simulink model "UberSpurs"  (R2015b)
settings: Solver=VariableStepAuto  StartTime=0.0  StopTime=5000  RelTol=1e-3
libraries: simulink x54
(part 5 of 6)

== system UberSpurs/spur3WorkCell/route2Channel16 ==
  serverAvailable : Inport
  Constant : Constant  Value=16
  Get Attribute : GetAttribute  AttributeName=Channel|FillTime  AttributeMissing=Error|Error  AttributeDefaultValue=1|1  AttributeTreatAsVector=1|1  AttributeSendTiming=After entity departure|After entity departure  EvaluatedDefaultAttributeValue={ [];[]}
      settings: OutputPortMap=o1,o2
  RoutingControlActuator : OutputSwitch  NumberOutputPorts=2  SwitchingCriterion=From signal port p  InitialConditionsOpt=on
  RoutingControlBehavior : Stateflow chart  TreatAsAtomicUnit=on
  Single Server1 : SingleServer  ServiceTime=0
  toChannel : PMIOPort  Port=1  Side=Right
  fromMHS : PMIOPort  Port=2  Side=Left
  toMHS : PMIOPort  Port=3  Side=Right
  wires:
  RoutingControlBehavior/1(route) -> RoutingControlActuator/1
  Constant/1 -> RoutingControlBehavior/2(channel)
  Get Attribute/1 -> RoutingControlBehavior/1(entityChannel)
  serverAvailable/1 -> RoutingControlBehavior/3(serverAvailable)
  Get Attribute/2 -> RoutingControlBehavior/4(FillTime)
  connections:
  RoutingControlActuator/RConn2 -- toMHS/RConn1
  Get Attribute/RConn1 -- Single Server1/LConn1
  fromMHS/RConn1 -- Get Attribute/LConn1
  toChannel/RConn1 -- RoutingControlActuator/RConn1
  Single Server1/RConn1 -- RoutingControlActuator/LConn1

== system UberSpurs/spur3WorkCell/route2Channel17 ==
  serverAvailable : Inport
  Constant : Constant  Value=17
  Get Attribute : GetAttribute  AttributeName=Channel|FillTime  AttributeMissing=Error|Error  AttributeDefaultValue=1|1  AttributeTreatAsVector=1|1  AttributeSendTiming=After entity departure|After entity departure  EvaluatedDefaultAttributeValue={ [];[]}
      settings: OutputPortMap=o1,o2
  RoutingControlActuator : OutputSwitch  NumberOutputPorts=2  SwitchingCriterion=From signal port p  InitialConditionsOpt=on
  RoutingControlBehavior : Stateflow chart  TreatAsAtomicUnit=on
  Single Server1 : SingleServer  ServiceTime=0
  toChannel : PMIOPort  Port=1  Side=Right
  fromMHS : PMIOPort  Port=2  Side=Left
  toMHS : PMIOPort  Port=3  Side=Right
  wires:
  RoutingControlBehavior/1(route) -> RoutingControlActuator/1
  Constant/1 -> RoutingControlBehavior/2(channel)
  Get Attribute/1 -> RoutingControlBehavior/1(entityChannel)
  serverAvailable/1 -> RoutingControlBehavior/3(serverAvailable)
  Get Attribute/2 -> RoutingControlBehavior/4(FillTime)
  connections:
  RoutingControlActuator/RConn2 -- toMHS/RConn1
  Get Attribute/RConn1 -- Single Server1/LConn1
  fromMHS/RConn1 -- Get Attribute/LConn1
  toChannel/RConn1 -- RoutingControlActuator/RConn1
  Single Server1/RConn1 -- RoutingControlActuator/LConn1

== system UberSpurs/spur3WorkCell/route2Channel18 ==
  serverAvailable : Inport
  Constant : Constant  Value=18
  Get Attribute : GetAttribute  AttributeName=Channel|FillTime  AttributeMissing=Error|Error  AttributeDefaultValue=1|1  AttributeTreatAsVector=1|1  AttributeSendTiming=After entity departure|After entity departure  EvaluatedDefaultAttributeValue={ [];[]}
      settings: OutputPortMap=o1,o2
  RoutingControlActuator : OutputSwitch  NumberOutputPorts=2  SwitchingCriterion=From signal port p  InitialConditionsOpt=on
  RoutingControlBehavior : Stateflow chart  TreatAsAtomicUnit=on
  Single Server1 : SingleServer  ServiceTime=0
  toChannel : PMIOPort  Port=1  Side=Right
  fromMHS : PMIOPort  Port=2  Side=Left
  toMHS : PMIOPort  Port=3  Side=Right
  wires:
  RoutingControlBehavior/1(route) -> RoutingControlActuator/1
  Constant/1 -> RoutingControlBehavior/2(channel)
  Get Attribute/1 -> RoutingControlBehavior/1(entityChannel)
  serverAvailable/1 -> RoutingControlBehavior/3(serverAvailable)
  Get Attribute/2 -> RoutingControlBehavior/4(FillTime)
  connections:
  RoutingControlActuator/RConn2 -- toMHS/RConn1
  Get Attribute/RConn1 -- Single Server1/LConn1
  fromMHS/RConn1 -- Get Attribute/LConn1
  toChannel/RConn1 -- RoutingControlActuator/RConn1
  Single Server1/RConn1 -- RoutingControlActuator/LConn1

== system UberSpurs/spur3WorkCell/route2Channel2 ==
  serverAvailable : Inport
  Constant : Constant  Value=2
  Get Attribute : GetAttribute  AttributeName=Channel|FillTime  AttributeMissing=Error|Error  AttributeDefaultValue=1|1  AttributeTreatAsVector=1|1  AttributeSendTiming=After entity departure|After entity departure  EvaluatedDefaultAttributeValue={ [];[]}
      settings: OutputPortMap=o1,o2
  RoutingControlActuator : OutputSwitch  NumberOutputPorts=2  SwitchingCriterion=From signal port p  InitialConditionsOpt=on
  RoutingControlBehavior : Stateflow chart  TreatAsAtomicUnit=on
  Single Server1 : SingleServer  ServiceTime=0
  toChannel : PMIOPort  Port=1  Side=Right
  fromMHS : PMIOPort  Port=2  Side=Left
  toMHS : PMIOPort  Port=3  Side=Right
  wires:
  RoutingControlBehavior/1(route) -> RoutingControlActuator/1
  Constant/1 -> RoutingControlBehavior/2(channel)
  Get Attribute/1 -> RoutingControlBehavior/1(entityChannel)
  serverAvailable/1 -> RoutingControlBehavior/3(serverAvailable)
  Get Attribute/2 -> RoutingControlBehavior/4(FillTime)
  connections:
  RoutingControlActuator/RConn2 -- toMHS/RConn1
  Get Attribute/RConn1 -- Single Server1/LConn1
  fromMHS/RConn1 -- Get Attribute/LConn1
  toChannel/RConn1 -- RoutingControlActuator/RConn1
  Single Server1/RConn1 -- RoutingControlActuator/LConn1

== system UberSpurs/spur3WorkCell/route2Channel3 ==
  serverAvailable : Inport
  Constant : Constant  Value=3
  Get Attribute : GetAttribute  AttributeName=Channel|FillTime  AttributeMissing=Error|Error  AttributeDefaultValue=1|1  AttributeTreatAsVector=1|1  AttributeSendTiming=After entity departure|After entity departure  EvaluatedDefaultAttributeValue={ [];[]}
      settings: OutputPortMap=o1,o2
  RoutingControlActuator : OutputSwitch  NumberOutputPorts=2  SwitchingCriterion=From signal port p  InitialConditionsOpt=on
  RoutingControlBehavior : Stateflow chart  TreatAsAtomicUnit=on
  Single Server1 : SingleServer  ServiceTime=0
  toChannel : PMIOPort  Port=1  Side=Right
  fromMHS : PMIOPort  Port=2  Side=Left
  toMHS : PMIOPort  Port=3  Side=Right
  wires:
  RoutingControlBehavior/1(route) -> RoutingControlActuator/1
  Constant/1 -> RoutingControlBehavior/2(channel)
  Get Attribute/1 -> RoutingControlBehavior/1(entityChannel)
  serverAvailable/1 -> RoutingControlBehavior/3(serverAvailable)
  Get Attribute/2 -> RoutingControlBehavior/4(FillTime)
  connections:
  RoutingControlActuator/RConn2 -- toMHS/RConn1
  Get Attribute/RConn1 -- Single Server1/LConn1
  fromMHS/RConn1 -- Get Attribute/LConn1
  toChannel/RConn1 -- RoutingControlActuator/RConn1
  Single Server1/RConn1 -- RoutingControlActuator/LConn1

== system UberSpurs/spur3WorkCell/route2Channel4 ==
  serverAvailable : Inport
  Constant : Constant  Value=4
  Get Attribute : GetAttribute  AttributeName=Channel|FillTime  AttributeMissing=Error|Error  AttributeDefaultValue=1|1  AttributeTreatAsVector=1|1  AttributeSendTiming=After entity departure|After entity departure  EvaluatedDefaultAttributeValue={ [];[]}
      settings: OutputPortMap=o1,o2
  RoutingControlActuator : OutputSwitch  NumberOutputPorts=2  SwitchingCriterion=From signal port p  InitialConditionsOpt=on
  RoutingControlBehavior : Stateflow chart  TreatAsAtomicUnit=on
  Single Server1 : SingleServer  ServiceTime=0
  toChannel : PMIOPort  Port=1  Side=Right
  fromMHS : PMIOPort  Port=2  Side=Left
  toMHS : PMIOPort  Port=3  Side=Right
  wires:
  RoutingControlBehavior/1(route) -> RoutingControlActuator/1
  Constant/1 -> RoutingControlBehavior/2(channel)
  Get Attribute/1 -> RoutingControlBehavior/1(entityChannel)
  serverAvailable/1 -> RoutingControlBehavior/3(serverAvailable)
  Get Attribute/2 -> RoutingControlBehavior/4(FillTime)
  connections:
  RoutingControlActuator/RConn2 -- toMHS/RConn1
  Get Attribute/RConn1 -- Single Server1/LConn1
  fromMHS/RConn1 -- Get Attribute/LConn1
  toChannel/RConn1 -- RoutingControlActuator/RConn1
  Single Server1/RConn1 -- RoutingControlActuator/LConn1

== system UberSpurs/spur3WorkCell/route2Channel5 ==
  serverAvailable : Inport
  Constant : Constant  Value=5
  Get Attribute : GetAttribute  AttributeName=Channel|FillTime  AttributeMissing=Error|Error  AttributeDefaultValue=1|1  AttributeTreatAsVector=1|1  AttributeSendTiming=After entity departure|After entity departure  EvaluatedDefaultAttributeValue={ [];[]}
      settings: OutputPortMap=o1,o2
  RoutingControlActuator : OutputSwitch  NumberOutputPorts=2  SwitchingCriterion=From signal port p  InitialConditionsOpt=on
  RoutingControlBehavior : Stateflow chart  TreatAsAtomicUnit=on
  Single Server1 : SingleServer  ServiceTime=0
  toChannel : PMIOPort  Port=1  Side=Right
  fromMHS : PMIOPort  Port=2  Side=Left
  toMHS : PMIOPort  Port=3  Side=Right
  wires:
  RoutingControlBehavior/1(route) -> RoutingControlActuator/1
  Constant/1 -> RoutingControlBehavior/2(channel)
  Get Attribute/1 -> RoutingControlBehavior/1(entityChannel)
  serverAvailable/1 -> RoutingControlBehavior/3(serverAvailable)
  Get Attribute/2 -> RoutingControlBehavior/4(FillTime)
  connections:
  RoutingControlActuator/RConn2 -- toMHS/RConn1
  Get Attribute/RConn1 -- Single Server1/LConn1
  fromMHS/RConn1 -- Get Attribute/LConn1
  toChannel/RConn1 -- RoutingControlActuator/RConn1
  Single Server1/RConn1 -- RoutingControlActuator/LConn1

== system UberSpurs/spur3WorkCell/route2Channel6 ==
  serverAvailable : Inport
  Constant : Constant  Value=6
  Get Attribute : GetAttribute  AttributeName=Channel|FillTime  AttributeMissing=Error|Error  AttributeDefaultValue=1|1  AttributeTreatAsVector=1|1  AttributeSendTiming=After entity departure|After entity departure  EvaluatedDefaultAttributeValue={ [];[]}
      settings: OutputPortMap=o1,o2
  RoutingControlActuator : OutputSwitch  NumberOutputPorts=2  SwitchingCriterion=From signal port p  InitialConditionsOpt=on
  RoutingControlBehavior : Stateflow chart  TreatAsAtomicUnit=on
  Single Server1 : SingleServer  ServiceTime=0
  toChannel : PMIOPort  Port=1  Side=Right
  fromMHS : PMIOPort  Port=2  Side=Left
  toMHS : PMIOPort  Port=3  Side=Right
  wires:
  RoutingControlBehavior/1(route) -> RoutingControlActuator/1
  Constant/1 -> RoutingControlBehavior/2(channel)
  Get Attribute/1 -> RoutingControlBehavior/1(entityChannel)
  serverAvailable/1 -> RoutingControlBehavior/3(serverAvailable)
  Get Attribute/2 -> RoutingControlBehavior/4(FillTime)
  connections:
  RoutingControlActuator/RConn2 -- toMHS/RConn1
  Get Attribute/RConn1 -- Single Server1/LConn1
  fromMHS/RConn1 -- Get Attribute/LConn1
  toChannel/RConn1 -- RoutingControlActuator/RConn1
  Single Server1/RConn1 -- RoutingControlActuator/LConn1

== system UberSpurs/spur3WorkCell/route2Channel7 ==
  serverAvailable : Inport
  Constant : Constant  Value=7
  Get Attribute : GetAttribute  AttributeName=Channel|FillTime  AttributeMissing=Error|Error  AttributeDefaultValue=1|1  AttributeTreatAsVector=1|1  AttributeSendTiming=After entity departure|After entity departure  EvaluatedDefaultAttributeValue={ [];[]}
      settings: OutputPortMap=o1,o2
  RoutingControlActuator : OutputSwitch  NumberOutputPorts=2  SwitchingCriterion=From signal port p  InitialConditionsOpt=on
  RoutingControlBehavior : Stateflow chart  TreatAsAtomicUnit=on
  Single Server1 : SingleServer  ServiceTime=0
  toChannel : PMIOPort  Port=1  Side=Right
  fromMHS : PMIOPort  Port=2  Side=Left
  toMHS : PMIOPort  Port=3  Side=Right
  wires:
  RoutingControlBehavior/1(route) -> RoutingControlActuator/1
  Constant/1 -> RoutingControlBehavior/2(channel)
  Get Attribute/1 -> RoutingControlBehavior/1(entityChannel)
  serverAvailable/1 -> RoutingControlBehavior/3(serverAvailable)
  Get Attribute/2 -> RoutingControlBehavior/4(FillTime)
  connections:
  RoutingControlActuator/RConn2 -- toMHS/RConn1
  Get Attribute/RConn1 -- Single Server1/LConn1
  fromMHS/RConn1 -- Get Attribute/LConn1
  toChannel/RConn1 -- RoutingControlActuator/RConn1
  Single Server1/RConn1 -- RoutingControlActuator/LConn1

== system UberSpurs/spur3WorkCell/route2Channel8 ==
  serverAvailable : Inport
  Constant : Constant  Value=8
  Get Attribute : GetAttribute  AttributeName=Channel|FillTime  AttributeMissing=Error|Error  AttributeDefaultValue=1|1  AttributeTreatAsVector=1|1  AttributeSendTiming=After entity departure|After entity departure  EvaluatedDefaultAttributeValue={ [];[]}
      settings: OutputPortMap=o1,o2
  RoutingControlActuator : OutputSwitch  NumberOutputPorts=2  SwitchingCriterion=From signal port p  InitialConditionsOpt=on
  RoutingControlBehavior : Stateflow chart  TreatAsAtomicUnit=on
  Single Server1 : SingleServer  ServiceTime=0
  toChannel : PMIOPort  Port=1  Side=Right
  fromMHS : PMIOPort  Port=2  Side=Left
  toMHS : PMIOPort  Port=3  Side=Right
  wires:
  RoutingControlBehavior/1(route) -> RoutingControlActuator/1
  Constant/1 -> RoutingControlBehavior/2(channel)
  Get Attribute/1 -> RoutingControlBehavior/1(entityChannel)
  serverAvailable/1 -> RoutingControlBehavior/3(serverAvailable)
  Get Attribute/2 -> RoutingControlBehavior/4(FillTime)
  connections:
  RoutingControlActuator/RConn2 -- toMHS/RConn1
  Get Attribute/RConn1 -- Single Server1/LConn1
  fromMHS/RConn1 -- Get Attribute/LConn1
  toChannel/RConn1 -- RoutingControlActuator/RConn1
  Single Server1/RConn1 -- RoutingControlActuator/LConn1

== system UberSpurs/spur3WorkCell/route2Channel9 ==
  serverAvailable : Inport
  Constant : Constant  Value=9
  Get Attribute : GetAttribute  AttributeName=Channel|FillTime  AttributeMissing=Error|Error  AttributeDefaultValue=1|1  AttributeTreatAsVector=1|1  AttributeSendTiming=After entity departure|After entity departure  EvaluatedDefaultAttributeValue={ [];[]}
      settings: OutputPortMap=o1,o2
  RoutingControlActuator : OutputSwitch  NumberOutputPorts=2  SwitchingCriterion=From signal port p  InitialConditionsOpt=on
  RoutingControlBehavior : Stateflow chart  TreatAsAtomicUnit=on
  Single Server1 : SingleServer  ServiceTime=0
  toChannel : PMIOPort  Port=1  Side=Right
  fromMHS : PMIOPort  Port=2  Side=Left
  toMHS : PMIOPort  Port=3  Side=Right
  wires:
  RoutingControlBehavior/1(route) -> RoutingControlActuator/1
  Constant/1 -> RoutingControlBehavior/2(channel)
  Get Attribute/1 -> RoutingControlBehavior/1(entityChannel)
  serverAvailable/1 -> RoutingControlBehavior/3(serverAvailable)
  Get Attribute/2 -> RoutingControlBehavior/4(FillTime)
  connections:
  RoutingControlActuator/RConn2 -- toMHS/RConn1
  Get Attribute/RConn1 -- Single Server1/LConn1
  fromMHS/RConn1 -- Get Attribute/LConn1
  toChannel/RConn1 -- RoutingControlActuator/RConn1
  Single Server1/RConn1 -- RoutingControlActuator/LConn1

== system UberSpurs/spur3WorkCell/route2recirculate ==
  verifyQueueLength : Inport
  Chart : Stateflow chart  TreatAsAtomicUnit=on
  Get Attribute : GetAttribute  AttributeName=FillTime  EvaluatedDefaultAttributeValue={ []}
      settings: OutputPortMap=o1
  Single Server1 : SingleServer  ServiceTime=0
  route2recirculate : OutputSwitch  NumberOutputPorts=2  SwitchingCriterion=From signal port p  InitialConditionsOpt=on
  recirculate : PMIOPort  Port=1  Side=Right
  fromMHS : PMIOPort  Port=2  Side=Left
  toverify : PMIOPort  Port=3  Side=Right
  wires:
  Chart/1(route) -> route2recirculate/1
  Get Attribute/1 -> Chart/1(FillTime)
  verifyQueueLength/1 -> Chart/2(verifyQueue)
  connections:
  Get Attribute/RConn1 -- Single Server1/LConn1
  fromMHS/RConn1 -- Get Attribute/LConn1
  Single Server1/RConn1 -- route2recirculate/LConn1
  route2recirculate/RConn2 -- toverify/RConn1
  route2recirculate/RConn1 -- recirculate/RConn1

== system UberSpurs/spur3WorkCell/verifyWorkstation ==
  Clock : Clock
  Set Attribute1 : SetAttribute  AttributeName=VerifyTime  AttributeFrom=Signal port  EvaluatedAttributeValue={ []}
  Timed to Event Sigal : TimedToEventSignal
  VerifyQueue : FIFOQueue  Capacity=1  StatNumberInBlock=on
      settings: OutputPortMap=o1
  VerifyServer : SingleServer  ServiceTimeFrom=Signal port t  ServiceTime=1.55
  processTime : EventBasedRandomNumber  Distribution=Arbitrary discrete  probVecDisc=[0 1]  Seed=7122
  vialOUT : PMIOPort  Port=1  Side=Left
  vialIN : PMIOPort  Port=2  Side=Right
  queueLength : Outport
  wires:
  processTime/1 -> VerifyServer/1
  Clock/1 -> Timed to Event Sigal/1
  Timed to Event Sigal/1 -> Set Attribute1/1
  VerifyQueue/1 -> queueLength/1
  connections:
  Set Attribute1/RConn1 -- vialOUT/RConn1
  VerifyQueue/RConn1 -- VerifyServer/LConn1
  VerifyQueue/LConn1 -- vialIN/RConn1
  Set Attribute1/LConn1 -- VerifyServer/RConn1

== stateflow chart UberSpurs/route2Spur1/routingControl ==
  (default) -> (junction 9) : % route2Spur
  (junction 9) -> (junction 10) [order 1] : [entitySpur == 1 & VerifyTime == 0]
  (junction 9) -> (junction 11) [order 2] : {route = 1;}
  (junction 10) -> (junction 12) : {route = 2;}
  (junction 12) -> (junction 11)
  (junction 11) -> (junction 13)
  data: entitySpur input; route output; VerifyTime input

== stateflow chart UberSpurs/spur1WorkCell/route2Channel2/RoutingControlBehavior ==
  (default) -> (junction 7) : % toChanel
  (junction 7) -> (junction 8) [order 1] : [entityChannel == channel & serverAvailable ==1 & FillTime == 0]
  (junction 7) -> (junction 9) [order 2] : {route = 2;}
  (junction 8) -> (junction 10) : {route = 1 ;}
  (junction 10) -> (junction 9)
  (junction 9) -> (junction 11)
  data: entityChannel input; channel input; route output; serverAvailable input; FillTime input

== stateflow chart UberSpurs/spur1WorkCell/route2Channel1/RoutingControlBehavior ==
  (default) -> (junction 7) : % toChanel
  (junction 7) -> (junction 8) [order 1] : [entityChannel == channel & serverAvailable ==1 & FillTime == 0]
  (junction 7) -> (junction 9) [order 2] : {route = 2;}
  (junction 8) -> (junction 10) : {route = 1 ;}
  (junction 10) -> (junction 9)
  (junction 9) -> (junction 11)
  data: entityChannel input; channel input; route output; serverAvailable input; FillTime input

== stateflow chart UberSpurs/spur1WorkCell/route2Channel3/RoutingControlBehavior ==
  (default) -> (junction 7) : % toChanel
  (junction 7) -> (junction 8) [order 1] : [entityChannel == channel & serverAvailable ==1 & FillTime == 0]
  (junction 7) -> (junction 9) [order 2] : {route = 2;}
  (junction 8) -> (junction 10) : {route = 1 ;}
  (junction 10) -> (junction 9)
  (junction 9) -> (junction 11)
  data: entityChannel input; channel input; route output; serverAvailable input; FillTime input

== stateflow chart UberSpurs/spur1WorkCell/route2Channel4/RoutingControlBehavior ==
  (default) -> (junction 7) : % toChanel
  (junction 7) -> (junction 8) [order 1] : [entityChannel == channel & serverAvailable ==1 & FillTime == 0]
  (junction 7) -> (junction 9) [order 2] : {route = 2;}
  (junction 8) -> (junction 10) : {route = 1 ;}
  (junction 10) -> (junction 9)
  (junction 9) -> (junction 11)
  data: entityChannel input; channel input; route output; serverAvailable input; FillTime input

== stateflow chart UberSpurs/spur1WorkCell/route2Channel5/RoutingControlBehavior ==
  (default) -> (junction 7) : % toChanel
  (junction 7) -> (junction 8) [order 1] : [entityChannel == channel & serverAvailable ==1 & FillTime == 0]
  (junction 7) -> (junction 9) [order 2] : {route = 2;}
  (junction 8) -> (junction 10) : {route = 1 ;}
  (junction 10) -> (junction 9)
  (junction 9) -> (junction 11)
  data: entityChannel input; channel input; route output; serverAvailable input; FillTime input

== stateflow chart UberSpurs/spur1WorkCell/route2Channel6/RoutingControlBehavior ==
  (default) -> (junction 7) : % toChanel
  (junction 7) -> (junction 8) [order 1] : [entityChannel == channel & serverAvailable ==1 & FillTime == 0]
  (junction 7) -> (junction 9) [order 2] : {route = 2;}
  (junction 8) -> (junction 10) : {route = 1 ;}
  (junction 10) -> (junction 9)
  (junction 9) -> (junction 11)
  data: entityChannel input; channel input; route output; serverAvailable input; FillTime input

== stateflow chart UberSpurs/spur1WorkCell/route2Channel7/RoutingControlBehavior ==
  (default) -> (junction 7) : % toChanel
  (junction 7) -> (junction 8) [order 1] : [entityChannel == channel & serverAvailable ==1 & FillTime == 0]
  (junction 7) -> (junction 9) [order 2] : {route = 2;}
  (junction 8) -> (junction 10) : {route = 1 ;}
  (junction 10) -> (junction 9)
  (junction 9) -> (junction 11)
  data: entityChannel input; channel input; route output; serverAvailable input; FillTime input

== stateflow chart UberSpurs/spur1WorkCell/route2Channel8/RoutingControlBehavior ==
  (default) -> (junction 7) : % toChanel
  (junction 7) -> (junction 8) [order 1] : [entityChannel == channel & serverAvailable ==1 & FillTime == 0]
  (junction 7) -> (junction 9) [order 2] : {route = 2;}
  (junction 8) -> (junction 10) : {route = 1 ;}
  (junction 10) -> (junction 9)
  (junction 9) -> (junction 11)
  data: entityChannel input; channel input; route output; serverAvailable input; FillTime input

== stateflow chart UberSpurs/spur1WorkCell/route2Channel9/RoutingControlBehavior ==
  (default) -> (junction 7) : % toChanel
  (junction 7) -> (junction 8) [order 1] : [entityChannel == channel & serverAvailable ==1 & FillTime == 0]
  (junction 7) -> (junction 9) [order 2] : {route = 2;}
  (junction 8) -> (junction 10) : {route = 1 ;}
  (junction 10) -> (junction 9)
  (junction 9) -> (junction 11)
  data: entityChannel input; channel input; route output; serverAvailable input; FillTime input

== stateflow chart UberSpurs/spur1WorkCell/route2recirculate/Chart ==
  (default) -> (junction 7) : % recirculate
  (junction 7) -> (junction 9) [order 1] : [FillTime>0]
  (junction 9) -> (junction 23) [order 1] : [verifyQueue<5]
  (junction 9) -> (junction 20) [order 2] : {route = 1;}
  (junction 7) -> (junction 8) [order 2] : {route = 1;}
  (junction 23) -> (junction 25) : {route = 2;}
  (junction 20) -> (junction 8)
  (junction 25) -> (junction 20)
  (junction 8) -> (junction 11)
  data: FillTime input; route output; verifyQueue input

== stateflow chart UberSpurs/orderRelease/AdmissionControlBehavior ==
  state dispatchOn
    during:
    admission = 1;
  state spursFull
    during:
    admission = 0;
  state labelFull
    during:
    admission = 0;
  (default) -> dispatchOn
  labelFull -> dispatchOn : [WIPlabel <10]
  dispatchOn -> spursFull [order 2] : [WIP>64]
  dispatchOn -> labelFull [order 1] : [WIPlabel == 45]
  spursFull -> dispatchOn : [WIP <=64]
  data: WIP input; admission output; WIPlabel input

== stateflow chart UberSpurs/spur1WorkCell/route2Channel10/RoutingControlBehavior ==
  (default) -> (junction 7) : % toChanel
  (junction 7) -> (junction 8) [order 1] : [entityChannel == channel & serverAvailable ==1 & FillTime == 0]
  (junction 7) -> (junction 9) [order 2] : {route = 2;}
  (junction 8) -> (junction 10) : {route = 1 ;}
  (junction 10) -> (junction 9)
  (junction 9) -> (junction 11)
  data: entityChannel input; channel input; route output; serverAvailable input; FillTime input

== stateflow chart UberSpurs/spur1WorkCell/route2Channel11/RoutingControlBehavior ==
  (default) -> (junction 7) : % toChanel
  (junction 7) -> (junction 8) [order 1] : [entityChannel == channel & serverAvailable ==1 & FillTime == 0]
  (junction 7) -> (junction 9) [order 2] : {route = 2;}
  (junction 8) -> (junction 10) : {route = 1 ;}
  (junction 10) -> (junction 9)
  (junction 9) -> (junction 11)
  data: entityChannel input; channel input; route output; serverAvailable input; FillTime input

== stateflow chart UberSpurs/spur1WorkCell/route2Channel12/RoutingControlBehavior ==
  (default) -> (junction 7) : % toChanel
  (junction 7) -> (junction 8) [order 1] : [entityChannel == channel & serverAvailable ==1 & FillTime == 0]
  (junction 7) -> (junction 9) [order 2] : {route = 2;}
  (junction 8) -> (junction 10) : {route = 1 ;}
  (junction 10) -> (junction 9)
  (junction 9) -> (junction 11)
  data: entityChannel input; channel input; route output; serverAvailable input; FillTime input

== stateflow chart UberSpurs/spur1WorkCell/route2Channel13/RoutingControlBehavior ==
  (default) -> (junction 7) : % toChanel
  (junction 7) -> (junction 8) [order 1] : [entityChannel == channel & serverAvailable ==1 & FillTime == 0]
  (junction 7) -> (junction 9) [order 2] : {route = 2;}
  (junction 8) -> (junction 10) : {route = 1 ;}
  (junction 10) -> (junction 9)
  (junction 9) -> (junction 11)
  data: entityChannel input; channel input; route output; serverAvailable input; FillTime input

== stateflow chart UberSpurs/spur1WorkCell/route2Channel14/RoutingControlBehavior ==
  (default) -> (junction 7) : % toChanel
  (junction 7) -> (junction 8) [order 1] : [entityChannel == channel & serverAvailable ==1 & FillTime == 0]
  (junction 7) -> (junction 9) [order 2] : {route = 2;}
  (junction 8) -> (junction 10) : {route = 1 ;}
  (junction 10) -> (junction 9)
  (junction 9) -> (junction 11)
  data: entityChannel input; channel input; route output; serverAvailable input; FillTime input

== stateflow chart UberSpurs/spur1WorkCell/route2Channel15/RoutingControlBehavior ==
  (default) -> (junction 7) : % toChanel
  (junction 7) -> (junction 8) [order 1] : [entityChannel == channel & serverAvailable ==1 & FillTime == 0]
  (junction 7) -> (junction 9) [order 2] : {route = 2;}
  (junction 8) -> (junction 10) : {route = 1 ;}
  (junction 10) -> (junction 9)
  (junction 9) -> (junction 11)
  data: entityChannel input; channel input; route output; serverAvailable input; FillTime input

== stateflow chart UberSpurs/spur1WorkCell/route2Channel16/RoutingControlBehavior ==
  (default) -> (junction 7) : % toChanel
  (junction 7) -> (junction 8) [order 1] : [entityChannel == channel & serverAvailable ==1 & FillTime == 0]
  (junction 7) -> (junction 9) [order 2] : {route = 2;}
  (junction 8) -> (junction 10) : {route = 1 ;}
  (junction 10) -> (junction 9)
  (junction 9) -> (junction 11)
  data: entityChannel input; channel input; route output; serverAvailable input; FillTime input

== stateflow chart UberSpurs/spur1WorkCell/route2Channel17/RoutingControlBehavior ==
  (default) -> (junction 7) : % toChanel
  (junction 7) -> (junction 8) [order 1] : [entityChannel == channel & serverAvailable ==1 & FillTime == 0]
  (junction 7) -> (junction 9) [order 2] : {route = 2;}
  (junction 8) -> (junction 10) : {route = 1 ;}
  (junction 10) -> (junction 9)
  (junction 9) -> (junction 11)
  data: entityChannel input; channel input; route output; serverAvailable input; FillTime input

== stateflow chart UberSpurs/spur1WorkCell/route2Channel18/RoutingControlBehavior ==
  (default) -> (junction 7) : % toChanel
  (junction 7) -> (junction 8) [order 1] : [entityChannel == channel & serverAvailable ==1 & FillTime == 0]
  (junction 7) -> (junction 9) [order 2] : {route = 2;}
  (junction 8) -> (junction 10) : {route = 1 ;}
  (junction 10) -> (junction 9)
  (junction 9) -> (junction 11)
  data: entityChannel input; channel input; route output; serverAvailable input; FillTime input

== stateflow chart UberSpurs/route2bagger4/routingControl ==
  (default) -> (junction 9) : % route2Bagger
  (junction 9) -> (junction 10) [order 1] : [entityBagger == 4 & queueLength <=10]
  (junction 9) -> (junction 11) [order 2] : {route = 1;}
  (junction 10) -> (junction 12) : {route = 2;}
  (junction 12) -> (junction 11)
  (junction 11) -> (junction 13)
  data: entityBagger input; route output; queueLength input

== stateflow chart UberSpurs/route2bagger3/routingControl ==
  (default) -> (junction 9) : % route2Bagger
  (junction 9) -> (junction 10) [order 1] : [entityBagger == 3 & queueLength <=10]
  (junction 9) -> (junction 11) [order 2] : {route = 1;}
  (junction 10) -> (junction 12) : {route = 2;}
  (junction 12) -> (junction 11)
  (junction 11) -> (junction 13)
  data: entityBagger input; route output; queueLength input

== stateflow chart UberSpurs/route2bagger2/routingControl ==
  (default) -> (junction 9) : % route2Bagger
  (junction 9) -> (junction 10) [order 1] : [entityBagger == 2 & queueLength <=10]
  (junction 9) -> (junction 11) [order 2] : {route = 1;}
  (junction 10) -> (junction 12) : {route = 2;}
  (junction 12) -> (junction 11)
  (junction 11) -> (junction 13)
  data: entityBagger input; route output; queueLength input

== stateflow chart UberSpurs/route2bagger1/routingControl ==
  (default) -> (junction 9) : % route2Bagger
  (junction 9) -> (junction 10) [order 1] : [entityBagger == 1 & queueLength <= 10]
  (junction 9) -> (junction 11) [order 2] : {route = 1;}
  (junction 10) -> (junction 12) : {route = 2;}
  (junction 12) -> (junction 11)
  (junction 11) -> (junction 13)
  data: entityBagger input; route output; queueLength input

== stateflow chart UberSpurs/route2Spur2/routingControl ==
  (default) -> (junction 9) : % route2Spur
  (junction 9) -> (junction 10) [order 1] : [entitySpur == 2 & VerifyTime == 0]
  (junction 9) -> (junction 11) [order 2] : {route = 1;}
  (junction 10) -> (junction 12) : {route = 2;}
  (junction 12) -> (junction 11)
  (junction 11) -> (junction 13)
  data: entitySpur input; route output; VerifyTime input

== stateflow chart UberSpurs/spur2WorkCell/route2Channel1/RoutingControlBehavior ==
  (default) -> (junction 7) : % toChanel
  (junction 7) -> (junction 8) [order 1] : [entityChannel == channel & serverAvailable ==1 & FillTime == 0]
  (junction 7) -> (junction 9) [order 2] : {route = 2;}
  (junction 8) -> (junction 10) : {route = 1 ;}
  (junction 10) -> (junction 9)
  (junction 9) -> (junction 11)
  data: entityChannel input; channel input; route output; serverAvailable input; FillTime input

== stateflow chart UberSpurs/spur2WorkCell/route2Channel10/RoutingControlBehavior ==
  (default) -> (junction 7) : % toChanel
  (junction 7) -> (junction 8) [order 1] : [entityChannel == channel & serverAvailable ==1 & FillTime == 0]
  (junction 7) -> (junction 9) [order 2] : {route = 2;}
  (junction 8) -> (junction 10) : {route = 1 ;}
  (junction 10) -> (junction 9)
  (junction 9) -> (junction 11)
  data: entityChannel input; channel input; route output; serverAvailable input; FillTime input

== stateflow chart UberSpurs/spur2WorkCell/route2Channel11/RoutingControlBehavior ==
  (default) -> (junction 7) : % toChanel
  (junction 7) -> (junction 8) [order 1] : [entityChannel == channel & serverAvailable ==1 & FillTime == 0]
  (junction 7) -> (junction 9) [order 2] : {route = 2;}
  (junction 8) -> (junction 10) : {route = 1 ;}
  (junction 10) -> (junction 9)
  (junction 9) -> (junction 11)
  data: entityChannel input; channel input; route output; serverAvailable input; FillTime input

== stateflow chart UberSpurs/spur2WorkCell/route2Channel12/RoutingControlBehavior ==
  (default) -> (junction 7) : % toChanel
  (junction 7) -> (junction 8) [order 1] : [entityChannel == channel & serverAvailable ==1 & FillTime == 0]
  (junction 7) -> (junction 9) [order 2] : {route = 2;}
  (junction 8) -> (junction 10) : {route = 1 ;}
  (junction 10) -> (junction 9)
  (junction 9) -> (junction 11)
  data: entityChannel input; channel input; route output; serverAvailable input; FillTime input

== stateflow chart UberSpurs/spur2WorkCell/route2Channel13/RoutingControlBehavior ==
  (default) -> (junction 7) : % toChanel
  (junction 7) -> (junction 8) [order 1] : [entityChannel == channel & serverAvailable ==1 & FillTime == 0]
  (junction 7) -> (junction 9) [order 2] : {route = 2;}
  (junction 8) -> (junction 10) : {route = 1 ;}
  (junction 10) -> (junction 9)
  (junction 9) -> (junction 11)
  data: entityChannel input; channel input; route output; serverAvailable input; FillTime input

== stateflow chart UberSpurs/spur2WorkCell/route2Channel14/RoutingControlBehavior ==
  (default) -> (junction 7) : % toChanel
  (junction 7) -> (junction 8) [order 1] : [entityChannel == channel & serverAvailable ==1 & FillTime == 0]
  (junction 7) -> (junction 9) [order 2] : {route = 2;}
  (junction 8) -> (junction 10) : {route = 1 ;}
  (junction 10) -> (junction 9)
  (junction 9) -> (junction 11)
  data: entityChannel input; channel input; route output; serverAvailable input; FillTime input

== stateflow chart UberSpurs/spur2WorkCell/route2Channel15/RoutingControlBehavior ==
  (default) -> (junction 7) : % toChanel
  (junction 7) -> (junction 8) [order 1] : [entityChannel == channel & serverAvailable ==1 & FillTime == 0]
  (junction 7) -> (junction 9) [order 2] : {route = 2;}
  (junction 8) -> (junction 10) : {route = 1 ;}
  (junction 10) -> (junction 9)
  (junction 9) -> (junction 11)
  data: entityChannel input; channel input; route output; serverAvailable input; FillTime input

== stateflow chart UberSpurs/spur2WorkCell/route2Channel16/RoutingControlBehavior ==
  (default) -> (junction 7) : % toChanel
  (junction 7) -> (junction 8) [order 1] : [entityChannel == channel & serverAvailable ==1 & FillTime == 0]
  (junction 7) -> (junction 9) [order 2] : {route = 2;}
  (junction 8) -> (junction 10) : {route = 1 ;}
  (junction 10) -> (junction 9)
  (junction 9) -> (junction 11)
  data: entityChannel input; channel input; route output; serverAvailable input; FillTime input

== stateflow chart UberSpurs/spur2WorkCell/route2Channel17/RoutingControlBehavior ==
  (default) -> (junction 7) : % toChanel
  (junction 7) -> (junction 8) [order 1] : [entityChannel == channel & serverAvailable ==1 & FillTime == 0]
  (junction 7) -> (junction 9) [order 2] : {route = 2;}
  (junction 8) -> (junction 10) : {route = 1 ;}
  (junction 10) -> (junction 9)
  (junction 9) -> (junction 11)
  data: entityChannel input; channel input; route output; serverAvailable input; FillTime input

== stateflow chart UberSpurs/spur2WorkCell/route2Channel18/RoutingControlBehavior ==
  (default) -> (junction 7) : % toChanel
  (junction 7) -> (junction 8) [order 1] : [entityChannel == channel & serverAvailable ==1 & FillTime == 0]
  (junction 7) -> (junction 9) [order 2] : {route = 2;}
  (junction 8) -> (junction 10) : {route = 1 ;}
  (junction 10) -> (junction 9)
  (junction 9) -> (junction 11)
  data: entityChannel input; channel input; route output; serverAvailable input; FillTime input

== stateflow chart UberSpurs/spur2WorkCell/route2Channel2/RoutingControlBehavior ==
  (default) -> (junction 7) : % toChanel
  (junction 7) -> (junction 8) [order 1] : [entityChannel == channel & serverAvailable ==1 & FillTime == 0]
  (junction 7) -> (junction 9) [order 2] : {route = 2;}
  (junction 8) -> (junction 10) : {route = 1 ;}
  (junction 10) -> (junction 9)
  (junction 9) -> (junction 11)
  data: entityChannel input; channel input; route output; serverAvailable input; FillTime input

== stateflow chart UberSpurs/spur2WorkCell/route2Channel3/RoutingControlBehavior ==
  (default) -> (junction 7) : % toChanel
  (junction 7) -> (junction 8) [order 1] : [entityChannel == channel & serverAvailable ==1 & FillTime == 0]
  (junction 7) -> (junction 9) [order 2] : {route = 2;}
  (junction 8) -> (junction 10) : {route = 1 ;}
  (junction 10) -> (junction 9)
  (junction 9) -> (junction 11)
  data: entityChannel input; channel input; route output; serverAvailable input; FillTime input

== stateflow chart UberSpurs/spur2WorkCell/route2Channel4/RoutingControlBehavior ==
  (default) -> (junction 7) : % toChanel
  (junction 7) -> (junction 8) [order 1] : [entityChannel == channel & serverAvailable ==1 & FillTime == 0]
  (junction 7) -> (junction 9) [order 2] : {route = 2;}
  (junction 8) -> (junction 10) : {route = 1 ;}
  (junction 10) -> (junction 9)
  (junction 9) -> (junction 11)
  data: entityChannel input; channel input; route output; serverAvailable input; FillTime input

== stateflow chart UberSpurs/spur2WorkCell/route2Channel5/RoutingControlBehavior ==
  (default) -> (junction 7) : % toChanel
  (junction 7) -> (junction 8) [order 1] : [entityChannel == channel & serverAvailable ==1 & FillTime == 0]
  (junction 7) -> (junction 9) [order 2] : {route = 2;}
  (junction 8) -> (junction 10) : {route = 1 ;}
  (junction 10) -> (junction 9)
  (junction 9) -> (junction 11)
  data: entityChannel input; channel input; route output; serverAvailable input; FillTime input

== stateflow chart UberSpurs/spur2WorkCell/route2Channel6/RoutingControlBehavior ==
  (default) -> (junction 7) : % toChanel
  (junction 7) -> (junction 8) [order 1] : [entityChannel == channel & serverAvailable ==1 & FillTime == 0]
  (junction 7) -> (junction 9) [order 2] : {route = 2;}
  (junction 8) -> (junction 10) : {route = 1 ;}
  (junction 10) -> (junction 9)
  (junction 9) -> (junction 11)
  data: entityChannel input; channel input; route output; serverAvailable input; FillTime input

== stateflow chart UberSpurs/spur2WorkCell/route2Channel7/RoutingControlBehavior ==
  (default) -> (junction 7) : % toChanel
  (junction 7) -> (junction 8) [order 1] : [entityChannel == channel & serverAvailable ==1 & FillTime == 0]
  (junction 7) -> (junction 9) [order 2] : {route = 2;}
  (junction 8) -> (junction 10) : {route = 1 ;}
  (junction 10) -> (junction 9)
  (junction 9) -> (junction 11)
  data: entityChannel input; channel input; route output; serverAvailable input; FillTime input

== stateflow chart UberSpurs/spur2WorkCell/route2Channel8/RoutingControlBehavior ==
  (default) -> (junction 7) : % toChanel
  (junction 7) -> (junction 8) [order 1] : [entityChannel == channel & serverAvailable ==1 & FillTime == 0]
  (junction 7) -> (junction 9) [order 2] : {route = 2;}
  (junction 8) -> (junction 10) : {route = 1 ;}
  (junction 10) -> (junction 9)
  (junction 9) -> (junction 11)
  data: entityChannel input; channel input; route output; serverAvailable input; FillTime input

== stateflow chart UberSpurs/spur2WorkCell/route2Channel9/RoutingControlBehavior ==
  (default) -> (junction 7) : % toChanel
  (junction 7) -> (junction 8) [order 1] : [entityChannel == channel & serverAvailable ==1 & FillTime == 0]
  (junction 7) -> (junction 9) [order 2] : {route = 2;}
  (junction 8) -> (junction 10) : {route = 1 ;}
  (junction 10) -> (junction 9)
  (junction 9) -> (junction 11)
  data: entityChannel input; channel input; route output; serverAvailable input; FillTime input

== stateflow chart UberSpurs/spur2WorkCell/route2recirculate/Chart ==
  (default) -> (junction 7) : % recirculate
  (junction 7) -> (junction 9) [order 1] : [FillTime>0]
  (junction 9) -> (junction 23) [order 1] : [verifyQueue<5]
  (junction 9) -> (junction 20) [order 2] : {route = 1;}
  (junction 7) -> (junction 8) [order 2] : {route = 1;}
  (junction 23) -> (junction 25) : {route = 2;}
  (junction 20) -> (junction 8)
  (junction 25) -> (junction 20)
  (junction 8) -> (junction 11)
  data: FillTime input; route output; verifyQueue input

== stateflow chart UberSpurs/route2Spur3/routingControl ==
  (default) -> (junction 9) : % route2Spur
  (junction 9) -> (junction 10) [order 1] : [entitySpur == 3 & VerifyTime == 0]
  (junction 9) -> (junction 11) [order 2] : {route = 1;}
  (junction 10) -> (junction 12) : {route = 2;}
  (junction 12) -> (junction 11)
  (junction 11) -> (junction 13)
  data: entitySpur input; route output; VerifyTime input

== stateflow chart UberSpurs/spur3WorkCell/route2Channel1/RoutingControlBehavior ==
  (default) -> (junction 7) : % toChanel
  (junction 7) -> (junction 8) [order 1] : [entityChannel == channel & serverAvailable ==1 & FillTime == 0]
  (junction 7) -> (junction 9) [order 2] : {route = 2;}
  (junction 8) -> (junction 10) : {route = 1 ;}
  (junction 10) -> (junction 9)
  (junction 9) -> (junction 11)
  data: entityChannel input; channel input; route output; serverAvailable input; FillTime input

== stateflow chart UberSpurs/spur3WorkCell/route2Channel10/RoutingControlBehavior ==
  (default) -> (junction 7) : % toChanel
  (junction 7) -> (junction 8) [order 1] : [entityChannel == channel & serverAvailable ==1 & FillTime == 0]
  (junction 7) -> (junction 9) [order 2] : {route = 2;}
  (junction 8) -> (junction 10) : {route = 1 ;}
  (junction 10) -> (junction 9)
  (junction 9) -> (junction 11)
  data: entityChannel input; channel input; route output; serverAvailable input; FillTime input

== stateflow chart UberSpurs/spur3WorkCell/route2Channel11/RoutingControlBehavior ==
  (default) -> (junction 7) : % toChanel
  (junction 7) -> (junction 8) [order 1] : [entityChannel == channel & serverAvailable ==1 & FillTime == 0]
  (junction 7) -> (junction 9) [order 2] : {route = 2;}
  (junction 8) -> (junction 10) : {route = 1 ;}
  (junction 10) -> (junction 9)
  (junction 9) -> (junction 11)
  data: entityChannel input; channel input; route output; serverAvailable input; FillTime input

== stateflow chart UberSpurs/spur3WorkCell/route2Channel12/RoutingControlBehavior ==
  (default) -> (junction 7) : % toChanel
  (junction 7) -> (junction 8) [order 1] : [entityChannel == channel & serverAvailable ==1 & FillTime == 0]
  (junction 7) -> (junction 9) [order 2] : {route = 2;}
  (junction 8) -> (junction 10) : {route = 1 ;}
  (junction 10) -> (junction 9)
  (junction 9) -> (junction 11)
  data: entityChannel input; channel input; route output; serverAvailable input; FillTime input

== stateflow chart UberSpurs/spur3WorkCell/route2Channel13/RoutingControlBehavior ==
  (default) -> (junction 7) : % toChanel
  (junction 7) -> (junction 8) [order 1] : [entityChannel == channel & serverAvailable ==1 & FillTime == 0]
  (junction 7) -> (junction 9) [order 2] : {route = 2;}
  (junction 8) -> (junction 10) : {route = 1 ;}
  (junction 10) -> (junction 9)
  (junction 9) -> (junction 11)
  data: entityChannel input; channel input; route output; serverAvailable input; FillTime input

== stateflow chart UberSpurs/spur3WorkCell/route2Channel14/RoutingControlBehavior ==
  (default) -> (junction 7) : % toChanel
  (junction 7) -> (junction 8) [order 1] : [entityChannel == channel & serverAvailable ==1 & FillTime == 0]
  (junction 7) -> (junction 9) [order 2] : {route = 2;}
  (junction 8) -> (junction 10) : {route = 1 ;}
  (junction 10) -> (junction 9)
  (junction 9) -> (junction 11)
  data: entityChannel input; channel input; route output; serverAvailable input; FillTime input

== stateflow chart UberSpurs/spur3WorkCell/route2Channel15/RoutingControlBehavior ==
  (default) -> (junction 7) : % toChanel
  (junction 7) -> (junction 8) [order 1] : [entityChannel == channel & serverAvailable ==1 & FillTime == 0]
  (junction 7) -> (junction 9) [order 2] : {route = 2;}
  (junction 8) -> (junction 10) : {route = 1 ;}
  (junction 10) -> (junction 9)
  (junction 9) -> (junction 11)
  data: entityChannel input; channel input; route output; serverAvailable input; FillTime input

== stateflow chart UberSpurs/spur3WorkCell/route2Channel16/RoutingControlBehavior ==
  (default) -> (junction 7) : % toChanel
  (junction 7) -> (junction 8) [order 1] : [entityChannel == channel & serverAvailable ==1 & FillTime == 0]
  (junction 7) -> (junction 9) [order 2] : {route = 2;}
  (junction 8) -> (junction 10) : {route = 1 ;}
  (junction 10) -> (junction 9)
  (junction 9) -> (junction 11)
  data: entityChannel input; channel input; route output; serverAvailable input; FillTime input

== stateflow chart UberSpurs/spur3WorkCell/route2Channel17/RoutingControlBehavior ==
  (default) -> (junction 7) : % toChanel
  (junction 7) -> (junction 8) [order 1] : [entityChannel == channel & serverAvailable ==1 & FillTime == 0]
  (junction 7) -> (junction 9) [order 2] : {route = 2;}
  (junction 8) -> (junction 10) : {route = 1 ;}
  (junction 10) -> (junction 9)
  (junction 9) -> (junction 11)
  data: entityChannel input; channel input; route output; serverAvailable input; FillTime input

== stateflow chart UberSpurs/spur3WorkCell/route2Channel18/RoutingControlBehavior ==
  (default) -> (junction 7) : % toChanel
  (junction 7) -> (junction 8) [order 1] : [entityChannel == channel & serverAvailable ==1 & FillTime == 0]
  (junction 7) -> (junction 9) [order 2] : {route = 2;}
  (junction 8) -> (junction 10) : {route = 1 ;}
  (junction 10) -> (junction 9)
  (junction 9) -> (junction 11)
  data: entityChannel input; channel input; route output; serverAvailable input; FillTime input

== stateflow chart UberSpurs/spur3WorkCell/route2Channel2/RoutingControlBehavior ==
  (default) -> (junction 7) : % toChanel
  (junction 7) -> (junction 8) [order 1] : [entityChannel == channel & serverAvailable ==1 & FillTime == 0]
  (junction 7) -> (junction 9) [order 2] : {route = 2;}
  (junction 8) -> (junction 10) : {route = 1 ;}
  (junction 10) -> (junction 9)
  (junction 9) -> (junction 11)
  data: entityChannel input; channel input; route output; serverAvailable input; FillTime input

== stateflow chart UberSpurs/spur3WorkCell/route2Channel3/RoutingControlBehavior ==
  (default) -> (junction 7) : % toChanel
  (junction 7) -> (junction 8) [order 1] : [entityChannel == channel & serverAvailable ==1 & FillTime == 0]
  (junction 7) -> (junction 9) [order 2] : {route = 2;}
  (junction 8) -> (junction 10) : {route = 1 ;}
  (junction 10) -> (junction 9)
  (junction 9) -> (junction 11)
  data: entityChannel input; channel input; route output; serverAvailable input; FillTime input

== stateflow chart UberSpurs/spur3WorkCell/route2Channel4/RoutingControlBehavior ==
  (default) -> (junction 7) : % toChanel
  (junction 7) -> (junction 8) [order 1] : [entityChannel == channel & serverAvailable ==1 & FillTime == 0]
  (junction 7) -> (junction 9) [order 2] : {route = 2;}
  (junction 8) -> (junction 10) : {route = 1 ;}
  (junction 10) -> (junction 9)
  (junction 9) -> (junction 11)
  data: entityChannel input; channel input; route output; serverAvailable input; FillTime input

== stateflow chart UberSpurs/spur3WorkCell/route2Channel5/RoutingControlBehavior ==
  (default) -> (junction 7) : % toChanel
  (junction 7) -> (junction 8) [order 1] : [entityChannel == channel & serverAvailable ==1 & FillTime == 0]
  (junction 7) -> (junction 9) [order 2] : {route = 2;}
  (junction 8) -> (junction 10) : {route = 1 ;}
  (junction 10) -> (junction 9)
  (junction 9) -> (junction 11)
  data: entityChannel input; channel input; route output; serverAvailable input; FillTime input

== stateflow chart UberSpurs/spur3WorkCell/route2Channel6/RoutingControlBehavior ==
  (default) -> (junction 7) : % toChanel
  (junction 7) -> (junction 8) [order 1] : [entityChannel == channel & serverAvailable ==1 & FillTime == 0]
  (junction 7) -> (junction 9) [order 2] : {route = 2;}
  (junction 8) -> (junction 10) : {route = 1 ;}
  (junction 10) -> (junction 9)
  (junction 9) -> (junction 11)
  data: entityChannel input; channel input; route output; serverAvailable input; FillTime input

== stateflow chart UberSpurs/spur3WorkCell/route2Channel7/RoutingControlBehavior ==
  (default) -> (junction 7) : % toChanel
  (junction 7) -> (junction 8) [order 1] : [entityChannel == channel & serverAvailable ==1 & FillTime == 0]
  (junction 7) -> (junction 9) [order 2] : {route = 2;}
  (junction 8) -> (junction 10) : {route = 1 ;}
  (junction 10) -> (junction 9)
  (junction 9) -> (junction 11)
  data: entityChannel input; channel input; route output; serverAvailable input; FillTime input

== stateflow chart UberSpurs/spur3WorkCell/route2Channel8/RoutingControlBehavior ==
  (default) -> (junction 7) : % toChanel
  (junction 7) -> (junction 8) [order 1] : [entityChannel == channel & serverAvailable ==1 & FillTime == 0]
  (junction 7) -> (junction 9) [order 2] : {route = 2;}
  (junction 8) -> (junction 10) : {route = 1 ;}
  (junction 10) -> (junction 9)
  (junction 9) -> (junction 11)
  data: entityChannel input; channel input; route output; serverAvailable input; FillTime input

== stateflow chart UberSpurs/spur3WorkCell/route2Channel9/RoutingControlBehavior ==
  (default) -> (junction 7) : % toChanel
  (junction 7) -> (junction 8) [order 1] : [entityChannel == channel & serverAvailable ==1 & FillTime == 0]
  (junction 7) -> (junction 9) [order 2] : {route = 2;}
  (junction 8) -> (junction 10) : {route = 1 ;}
  (junction 10) -> (junction 9)
  (junction 9) -> (junction 11)
  data: entityChannel input; channel input; route output; serverAvailable input; FillTime input

== stateflow chart UberSpurs/spur3WorkCell/route2recirculate/Chart ==
  (default) -> (junction 7) : % recirculate
  (junction 7) -> (junction 9) [order 1] : [FillTime>0]
  (junction 9) -> (junction 23) [order 1] : [verifyQueue<5]
  (junction 9) -> (junction 20) [order 2] : {route = 1;}
  (junction 7) -> (junction 8) [order 2] : {route = 1;}
  (junction 23) -> (junction 25) : {route = 2;}
  (junction 20) -> (junction 8)
  (junction 25) -> (junction 20)
  (junction 8) -> (junction 11)
  data: FillTime input; route output; verifyQueue input

== stateflow chart UberSpurs/route2Exception/exceptions ==
  (default) -> (junction 2) : %exceptions
  (junction 2) -> (junction 9) [order 1] : [exceptions==1]
  (junction 2) -> (junction 11) [order 2] : {route=1;}
  (junction 9) -> (junction 12) : {route=2;}
  (junction 12) -> (junction 11)
  (junction 11) -> (junction 16)
  data: exceptions input; route output

== stateflow chart UberSpurs/mergeOntoMainConveyor/mergeControl ==
  settings: executeAtInitialization=1
  state new
    during:
    merge = 0;
    recirculate = 0;
  state recirculate
    during:
    merge = 1;
    recirculate = 0;
  (default) -> new
  new -> recirculate : [recirculateQueue >= 10 ]
  recirculate -> new : [recirculateQueue < 6]
  data: recirculateQueue input; merge output =0; recirculate output =0
